simulink model "Arm_cobot"  (Simulink 8.3)
settings: Solver=ode1  StartTime=0.0  StopTime=inf  FixedStep=TA  RelTol=1e-3
PreLoadFcn:
  | startup
  | gui_starter
  | init_starter
PostLoadFcn:
  | init_check
InitFcn:
  | init_starter
undefined symbols (not defined in the file): alphaM, alphaT, Arm7ConLib, Arms2, baseOffset_x, baseOffset_y, baseOffset_z, betaM, betaT, cobotNa, cobotNb, D1, D2, D3, D4, D5, D6, D7, d_FTS_EE_L, d_FTS_EE_R, DD1, DD2, DD3, DD4, DD5, DD6, DD7, Do, Dp, EEL, EER, Fcal_L, Fcal_R, I1, I2, I3, I4, I5, I6, I7, IFL, IFR, impuls2rad_L, impuls2rad_R, Inert_L, Inert_R, KdC, KiC, Ko, Kp, KpC, LTool_L, LTool_R, mEE_L, mEE_R, Mo, Mp, P1, P2, P3 ... (+28)
libraries: sensoray x16, rtai_utilities x11, simulink x2, jr3lib x2, Interface x1
(part 2 of 3)

== system Arm_cobot/Left Arm/PD Joint Control  LEFT/PID Digital Derivative1 ==
  In1 : Inport
  Demux : Demux  Outputs=7
  Mux : Mux  Inputs=7
  PID + digital Derivative1 : Subsystem  AncestorBlock=|  mask(PID(2) Controller){P=P(1), I=I(1), D=D(1), N=N(1)}
      | Arm7lib/PID
      | Digital Derivative/PID +
      | digital Derivative2
      mask prompts: P "Proportional:"; I "Integral:"; D "Derivative:"; N "Derivative divisor(N):"
      mask help:
      | Enter Proportional(P), Integral(I), and Derivative(D) and divisor (N) terms.
      | P+I/s+Ds/(1/Ns+1)
      mask Help: This block implements a PID controller where parameters are entered for the Proportional, Integral and Derivative and divisor terms. Unmask this block to see how it works. The derivative term is implemented using an s/(s/N +1)  transfer function block. Making N large can create a "stiff" system.
      mask Display: disp('PID')
  PID + digital Derivative2 : Subsystem  AncestorBlock=|  mask(PID(2) Controller){P=P(3), I=I(3), D=D(3), N=N(3)}
      | Arm7lib/PID
      | Digital Derivative/PID +
      | digital Derivative2
      mask prompts: P "Proportional:"; I "Integral:"; D "Derivative:"; N "Derivative divisor(N):"
      mask help:
      | Enter Proportional(P), Integral(I), and Derivative(D) and divisor (N) terms.
      | P+I/s+Ds/(1/Ns+1)
      mask Help: This block implements a PID controller where parameters are entered for the Proportional, Integral and Derivative and divisor terms. Unmask this block to see how it works. The derivative term is implemented using an s/(s/N +1)  transfer function block. Making N large can create a "stiff" system.
      mask Display: disp('PID')
  PID + digital Derivative3 : Subsystem  AncestorBlock=|  mask(PID(2) Controller){P=P(2), I=I(2), D=D(2), N=N(2)}
      | Arm7lib/PID
      | Digital Derivative/PID +
      | digital Derivative2
      mask prompts: P "Proportional:"; I "Integral:"; D "Derivative:"; N "Derivative divisor(N):"
      mask help:
      | Enter Proportional(P), Integral(I), and Derivative(D) and divisor (N) terms.
      | P+I/s+Ds/(1/Ns+1)
      mask Help: This block implements a PID controller where parameters are entered for the Proportional, Integral and Derivative and divisor terms. Unmask this block to see how it works. The derivative term is implemented using an s/(s/N +1)  transfer function block. Making N large can create a "stiff" system.
      mask Display: disp('PID')
  PID + digital Derivative4 : Subsystem  AncestorBlock=|  mask(PID(2) Controller){P=P(4), I=I(4), D=D(4), N=N(4)}
      | Arm7lib/PID
      | Digital Derivative/PID +
      | digital Derivative2
      mask prompts: P "Proportional:"; I "Integral:"; D "Derivative:"; N "Derivative divisor(N):"
      mask help:
      | Enter Proportional(P), Integral(I), and Derivative(D) and divisor (N) terms.
      | P+I/s+Ds/(1/Ns+1)
      mask Help: This block implements a PID controller where parameters are entered for the Proportional, Integral and Derivative and divisor terms. Unmask this block to see how it works. The derivative term is implemented using an s/(s/N +1)  transfer function block. Making N large can create a "stiff" system.
      mask Display: disp('PID')
  PID + digital Derivative5 : Subsystem  AncestorBlock=|  mask(PID(2) Controller){P=P(5), I=I(5), D=D(5), N=N(5)}
      | Arm7lib/PID
      | Digital Derivative/PID +
      | digital Derivative2
      mask prompts: P "Proportional:"; I "Integral:"; D "Derivative:"; N "Derivative divisor(N):"
      mask help:
      | Enter Proportional(P), Integral(I), and Derivative(D) and divisor (N) terms.
      | P+I/s+Ds/(1/Ns+1)
      mask Help: This block implements a PID controller where parameters are entered for the Proportional, Integral and Derivative and divisor terms. Unmask this block to see how it works. The derivative term is implemented using an s/(s/N +1)  transfer function block. Making N large can create a "stiff" system.
      mask Display: disp('PID')
  PID + digital Derivative6 : Subsystem  AncestorBlock=|  mask(PID(2) Controller){P=P(6), I=I(6), D=D(6), N=N(6)}
      | Arm7lib/PID
      | Digital Derivative/PID +
      | digital Derivative2
      mask prompts: P "Proportional:"; I "Integral:"; D "Derivative:"; N "Derivative divisor(N):"
      mask help:
      | Enter Proportional(P), Integral(I), and Derivative(D) and divisor (N) terms.
      | P+I/s+Ds/(1/Ns+1)
      mask Help: This block implements a PID controller where parameters are entered for the Proportional, Integral and Derivative and divisor terms. Unmask this block to see how it works. The derivative term is implemented using an s/(s/N +1)  transfer function block. Making N large can create a "stiff" system.
      mask Display: disp('PID')
  PID + digital Derivative7 : Subsystem  AncestorBlock=|  mask(PID(2) Controller){P=P(7), I=I(7), D=D(7), N=N(7)}
      | Arm7lib/PID
      | Digital Derivative/PID +
      | digital Derivative2
      mask prompts: P "Proportional:"; I "Integral:"; D "Derivative:"; N "Derivative divisor(N):"
      mask help:
      | Enter Proportional(P), Integral(I), and Derivative(D) and divisor (N) terms.
      | P+I/s+Ds/(1/Ns+1)
      mask Help: This block implements a PID controller where parameters are entered for the Proportional, Integral and Derivative and divisor terms. Unmask this block to see how it works. The derivative term is implemented using an s/(s/N +1)  transfer function block. Making N large can create a "stiff" system.
      mask Display: disp('PID')
  Out1 : Outport
  wires:
  PID + digital Derivative7/1(Out_1) -> Mux/7
  PID + digital Derivative6/1(Out_1) -> Mux/6
  PID + digital Derivative5/1(Out_1) -> Mux/5
  PID + digital Derivative4/1(Out_1) -> Mux/4
  PID + digital Derivative2/1(Out_1) -> Mux/3
  PID + digital Derivative3/1(Out_1) -> Mux/2
  Demux/7 -> PID + digital Derivative7/1(In_1)
  Demux/6 -> PID + digital Derivative6/1(In_1)
  Demux/5 -> PID + digital Derivative5/1(In_1)
  Demux/4 -> PID + digital Derivative4/1(In_1)
  Demux/3 -> PID + digital Derivative2/1(In_1)
  Demux/2 -> PID + digital Derivative3/1(In_1)
  Mux/1 -> Out1/1
  PID + digital Derivative1/1(Out_1) -> Mux/1
  Demux/1 -> PID + digital Derivative1/1(In_1)
  In1/1 -> Demux/1

== system Arm_cobot/Left Arm/Switch between position control for Init position and regular controller/BackToInit1 ==
  JointAngles [rad] : Inport
  Clock : Clock
  "InitialJointAngles " : Constant  Value=qIL
  InitialPosition : S-Function  FunctionName=BackToInitJointSpace  EnableBusSupport=off
  Integrator : Integrator  InitialConditionSource=external
  Mux : Mux  Inputs=3
  Zeros : Constant  Value=zeros(1,7)
  q [rad] : Outport
  wires:
  Clock/1 -> Mux/3
  Mux/1 -> InitialPosition/1
  JointAngles [rad]/1 -> Integrator/2
  Zeros/1 -> Integrator/1
  Integrator/1 -> Mux/1
  InitialPosition/1 -> q [rad]/1
  "InitialJointAngles "/1 -> Mux/2

== system Arm_cobot/Right Arm/Feedforward/second  derivative ==
  q : Inport
  2ndDerivative3Points : MATLAB Function  TreatAsAtomicUnit=on
  Constant : Constant  Value=10*ones(1,7)
  Constant1 : Constant  Value=-10*ones(1,7)
  Memory : Memory
  Memory1 : Memory
  Rate Limiter Dynamic : simulink/Discontinuities/Rate Limiter Dynamic
  qDotDot : Outport
  wires:
  q/1 -> Memory/1, 2ndDerivative3Points/1(u0)
  Memory/1 -> Memory1/1, 2ndDerivative3Points/2(u1)
  Memory1/1 -> 2ndDerivative3Points/3(u2)
  Constant/1 -> Rate Limiter Dynamic/1
  Constant1/1 -> Rate Limiter Dynamic/3
  Rate Limiter Dynamic/1 -> qDotDot/1
  2ndDerivative3Points/1(y) -> Rate Limiter Dynamic/2

== system Arm_cobot/Right Arm/ForceControl/Subsystem ==
  In1 : Inport
  reset : Inport  Port=2
  Demux : Demux  Outputs=6
  Mux : Mux  Inputs=6
  PII : Subsystem  AncestorBlock=|  mask(PID(2) Controller){P=PF(1), I=IF(1), S=SF(1)}
      | Arm7lib/PID
      | Digital Derivative/PID +
      | digital Derivative2
      mask prompts: P "Proportional:"; I "Integral:"; S "Saturation:"
      mask help:
      | Enter Proportional(P), Integral(I), and Derivative(D) and divisor (N) terms.
      | P+I/s+Ds/(1/Ns+1)
      mask Help: This block implements a PID controller where parameters are entered for the Proportional, Integral and Derivative and divisor terms. Unmask this block to see how it works. The derivative term is implemented using an s/(s/N +1)  transfer function block. Making N large can create a "stiff" system.
      mask Display: disp('PI')
  PII1 : Subsystem  AncestorBlock=|  mask(PID(2) Controller){P=PF(2), I=IF(2), S=SF(2)}
      | Arm7lib/PID
      | Digital Derivative/PID +
      | digital Derivative2
      mask prompts: P "Proportional:"; I "Integral:"; S "Saturation:"
      mask help:
      | Enter Proportional(P), Integral(I), and Derivative(D) and divisor (N) terms.
      | P+I/s+Ds/(1/Ns+1)
      mask Help: This block implements a PID controller where parameters are entered for the Proportional, Integral and Derivative and divisor terms. Unmask this block to see how it works. The derivative term is implemented using an s/(s/N +1)  transfer function block. Making N large can create a "stiff" system.
      mask Display: disp('PI')
  PII2 : Subsystem  AncestorBlock=|  mask(PID(2) Controller){P=PF(3), I=IF(3), S=SF(3)}
      | Arm7lib/PID
      | Digital Derivative/PID +
      | digital Derivative2
      mask prompts: P "Proportional:"; I "Integral:"; S "Saturation:"
      mask help:
      | Enter Proportional(P), Integral(I), and Derivative(D) and divisor (N) terms.
      | P+I/s+Ds/(1/Ns+1)
      mask Help: This block implements a PID controller where parameters are entered for the Proportional, Integral and Derivative and divisor terms. Unmask this block to see how it works. The derivative term is implemented using an s/(s/N +1)  transfer function block. Making N large can create a "stiff" system.
      mask Display: disp('PI')
  PII3 : Subsystem  AncestorBlock=|  mask(PID(2) Controller){P=PF(4), I=IF(4), S=SF(4)}
      | Arm7lib/PID
      | Digital Derivative/PID +
      | digital Derivative2
      mask prompts: P "Proportional:"; I "Integral:"; S "Saturation:"
      mask help:
      | Enter Proportional(P), Integral(I), and Derivative(D) and divisor (N) terms.
      | P+I/s+Ds/(1/Ns+1)
      mask Help: This block implements a PID controller where parameters are entered for the Proportional, Integral and Derivative and divisor terms. Unmask this block to see how it works. The derivative term is implemented using an s/(s/N +1)  transfer function block. Making N large can create a "stiff" system.
      mask Display: disp('PI')
  PII4 : Subsystem  AncestorBlock=|  mask(PID(2) Controller){P=PF(5), I=IF(5), S=SF(5)}
      | Arm7lib/PID
      | Digital Derivative/PID +
      | digital Derivative2
      mask prompts: P "Proportional:"; I "Integral:"; S "Saturation:"
      mask help:
      | Enter Proportional(P), Integral(I), and Derivative(D) and divisor (N) terms.
      | P+I/s+Ds/(1/Ns+1)
      mask Help: This block implements a PID controller where parameters are entered for the Proportional, Integral and Derivative and divisor terms. Unmask this block to see how it works. The derivative term is implemented using an s/(s/N +1)  transfer function block. Making N large can create a "stiff" system.
      mask Display: disp('PI')
  PII5 : Subsystem  AncestorBlock=|  mask(PID(2) Controller){P=PF(6), I=IF(6), S=SF(6)}
      | Arm7lib/PID
      | Digital Derivative/PID +
      | digital Derivative2
      mask prompts: P "Proportional:"; I "Integral:"; S "Saturation:"
      mask help:
      | Enter Proportional(P), Integral(I), and Derivative(D) and divisor (N) terms.
      | P+I/s+Ds/(1/Ns+1)
      mask Help: This block implements a PID controller where parameters are entered for the Proportional, Integral and Derivative and divisor terms. Unmask this block to see how it works. The derivative term is implemented using an s/(s/N +1)  transfer function block. Making N large can create a "stiff" system.
      mask Display: disp('PI')
  Out1 : Outport
  wires:
  In1/1 -> Demux/1
  Demux/1 -> PII/1(In_1)
  Demux/2 -> PII1/1(In_1)
  Demux/3 -> PII2/1(In_1)
  Demux/5 -> PII4/1(In_1)
  PII/1(Out_1) -> Mux/1
  PII1/1(Out_1) -> Mux/2
  PII2/1(Out_1) -> Mux/3
  PII3/1(Out_1) -> Mux/4
  PII4/1(Out_1) -> Mux/5
  PII5/1(Out_1) -> Mux/6
  Mux/1 -> Out1/1
  Demux/6 -> PII5/1(In_1)
  reset/1 -> PII/2(reset), PII1/2(reset), PII2/2(reset), PII3/2(reset), PII5/2(reset), PII4/2(reset)
  Demux/4 -> PII3/1(In_1)

== system Arm_cobot/Right Arm/ForceControl/lowpass ==
  fLc : Inport
  Demux : Demux  Outputs=6
  Discrete Filter{,1..5} (6 alike) : DiscreteFilter  Numerator=[0.1 0.1 0.1 0.1 0.1 0.1 0.1 0.1 0.1 0.1]  Denominator=[1]
  Mux2 : Mux  Inputs=6
  Rate Transition3 : RateTransition  X0=-1
  smoothed : Outport
  wires:
  Discrete Filter/1 -> Mux2/1
  Demux/1 -> Discrete Filter/1
  Demux/2 -> Discrete Filter1/1
  Demux/3 -> Discrete Filter2/1
  Demux/4 -> Discrete Filter3/1
  Demux/5 -> Discrete Filter4/1
  Demux/6 -> Discrete Filter5/1
  Discrete Filter1/1 -> Mux2/2
  Discrete Filter3/1 -> Mux2/4
  Discrete Filter4/1 -> Mux2/5
  Discrete Filter5/1 -> Mux2/6
  Mux2/1 -> smoothed/1
  fLc/1 -> Rate Transition3/1
  Rate Transition3/1 -> Demux/1
  Discrete Filter2/1 -> Mux2/3

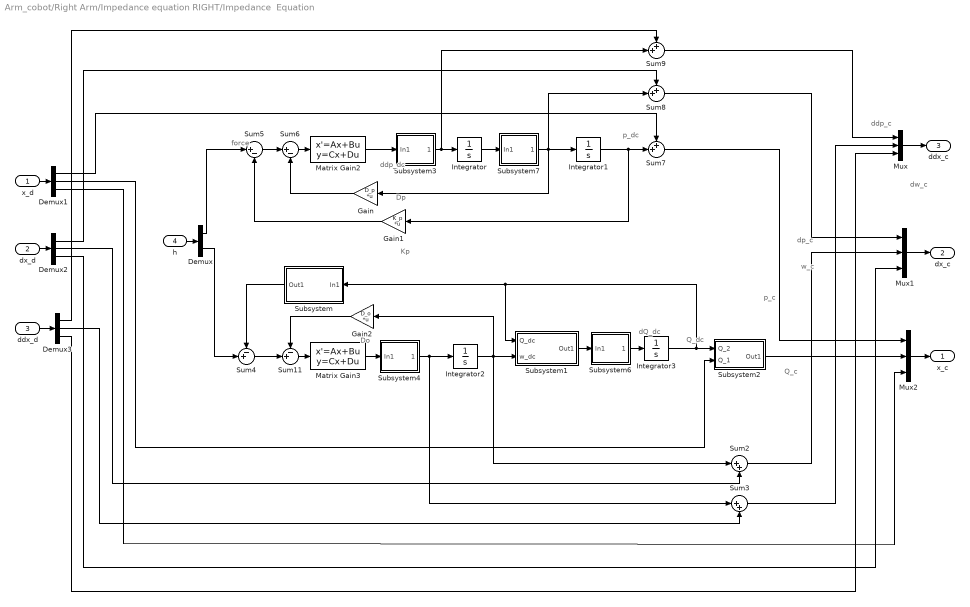
== system Arm_cobot/Right Arm/Impedance equation RIGHT/Impedance  Equation ==
  note: Do
  note: Dp
  note: Kp
  note: p_dc
  note: ddp_dc
  note: force
  note: p_c
  note: dp_c
  note: ddp_c
  note: dQ_dc
  note: Q_dc
  note: dw_c
  note: w_c
  note: Q_c
  x_d : Inport
  dx_d : Inport  Port=2
  ddx_d : Inport  Port=3
  h : Inport  Port=4
  Demux : Demux  Outputs=[3,3]
  Demux1 : Demux  Outputs=[3, 4, 1]
  Demux2 : Demux  Outputs=[3,3,1]
  Demux3 : Demux  Outputs=[3,3,1]
  Gain : Gain  Gain=D_p  Multiplication=Matrix(K*u)  OutDataTypeStr=Inherit: Same as input  ParamDataTypeStr=Inherit: Same as input
  Gain1 : Gain  Gain=K_p  Multiplication=Matrix(K*u)  OutDataTypeStr=Inherit: Same as input  ParamDataTypeStr=Inherit: Same as input
  Gain2 : Gain  Gain=D_o  Multiplication=Matrix(K*u)  OutDataTypeStr=Inherit: Same as input  ParamDataTypeStr=Inherit: Same as input
  Integrator : Integrator  InitialCondition=[0 0 0]
  Integrator1 : Integrator  InitialCondition=[0 0 0]
  Integrator2 : Integrator  InitialCondition=[0 0 0]
  Integrator3 : Integrator  InitialCondition=[1 0 0 0]
  Matrix Gain2 : StateSpace  A=[]  B=[]  C=[]  D=K  X0=0  mask(Matrix Gain){K=inv(M_p)}
      mask prompts: K "Gain matrix:"
      mask help: Matrix Gain.
      mask Help: Multiplies input vector by entered matrix to produce output vector (y=Au).
      mask Display: disp('inv(Mp)')
  Matrix Gain3 : StateSpace  A=[]  B=[]  C=[]  D=K  X0=0  mask(Matrix Gain){K=inv(M_o)}
      mask prompts: K "Gain matrix:"
      mask help: Matrix Gain.
      mask Help: Multiplies input vector by entered matrix to produce output vector (y=Au).
      mask Display: disp('inv(Mo)')
  Mux : Mux  Inputs=3
  Mux1 : Mux  Inputs=3
  Mux2 : Mux  Inputs=[3,4,1]
  Subsystem : Subsystem
      mask Display: disp('2*tr(E)*Ko')
  Subsystem1 : Subsystem
      mask Display: disp('Quaternion\n Propagation')
  Subsystem2 : Subsystem
      mask Display: disp('Qproduct')
  Subsystem3 : Subsystem
  Subsystem4 : Subsystem
  Subsystem6 : Subsystem
  Subsystem7 : Subsystem
  Sum11 : Sum  Inputs=-+|  SaturateOnIntegerOverflow=on  InputSameDT=on  OutDataTypeStr=Inherit: Same as first input
  Sum2 : Sum  Inputs=|++  SaturateOnIntegerOverflow=on  InputSameDT=on  OutDataTypeStr=Inherit: Same as first input
  Sum3 : Sum  Inputs=|++  SaturateOnIntegerOverflow=on  InputSameDT=on  OutDataTypeStr=Inherit: Same as first input
  Sum4 : Sum  Inputs=-+|  SaturateOnIntegerOverflow=on  InputSameDT=on  OutDataTypeStr=Inherit: Same as first input
  Sum5 : Sum  Inputs=|+-  SaturateOnIntegerOverflow=on  InputSameDT=on  OutDataTypeStr=Inherit: Same as first input
  Sum6 : Sum  Inputs=|+-  SaturateOnIntegerOverflow=on  InputSameDT=on  OutDataTypeStr=Inherit: Same as first input
  Sum7 : Sum  Inputs=++|  SaturateOnIntegerOverflow=on  InputSameDT=on  OutDataTypeStr=Inherit: Same as first input
  Sum8 : Sum  Inputs=++|  SaturateOnIntegerOverflow=on  InputSameDT=on  OutDataTypeStr=Inherit: Same as first input
  Sum9 : Sum  Inputs=++|  SaturateOnIntegerOverflow=on  InputSameDT=on  OutDataTypeStr=Inherit: Same as first input
  x_c : Outport
  dx_c : Outport  Port=2
  ddx_c : Outport  Port=3
  wires:
  Demux1/2 -> Subsystem2/2(Q_1)
  Subsystem2/1(Out1) -> Mux2/2
  Mux2/1 -> x_c/1
  Demux3/2 -> Sum3/2
  Demux3/3 -> Mux/3
  Mux1/1 -> dx_c/1
  Demux1/3 -> Mux2/3
  Demux2/3 -> Mux1/3
  Gain1/1 -> Sum5/2
  Gain/1 -> Sum6/2
  Subsystem1/1(Out1) -> Subsystem6/1(In1)
  Subsystem/1(Out1) -> Sum4/1
  Sum8/1 -> Mux1/1
  Sum6/1 -> Matrix Gain2/1
  Integrator1/1 -> Sum7/2, Gain1/1
  Sum5/1 -> Sum6/1
  Integrator/1 -> Subsystem7/1(In1)
  Integrator2/1 -> Subsystem1/2(w_dc), Gain2/1, Sum2/1
  Matrix Gain3/1 -> Subsystem4/1(In1)
  Sum2/1 -> Mux1/2
  h/1 -> Demux/1
  Sum9/1 -> Mux/1
  Mux/1 -> ddx_c/1
  Gain2/1 -> Sum11/1
  Sum11/1 -> Matrix Gain3/1
  Sum4/1 -> Sum11/2
  x_d/1 -> Demux1/1
  dx_d/1 -> Demux2/1
  ddx_d/1 -> Demux3/1
  Demux1/1 -> Sum7/1
  Demux2/2 -> Sum2/2
  Demux2/1 -> Sum8/1
  Demux3/1 -> Sum9/1
  Sum3/1 -> Mux/2
  Integrator3/1 -> Subsystem2/1(Q_2), Subsystem/1(In1), Subsystem1/1(Q_dc)
  Sum7/1 -> Mux2/1
  Demux/1 -> Sum5/1
  Demux/2 -> Sum4/2
  Subsystem3/1(Out1) -> Integrator/1, Sum9/2
  Matrix Gain2/1 -> Subsystem3/1(In1)
  Subsystem6/1(Out1) -> Integrator3/1
  Subsystem7/1(Out1) -> Sum8/2, Gain/1, Integrator1/1
  Subsystem4/1(Out1) -> Sum3/1, Integrator2/1

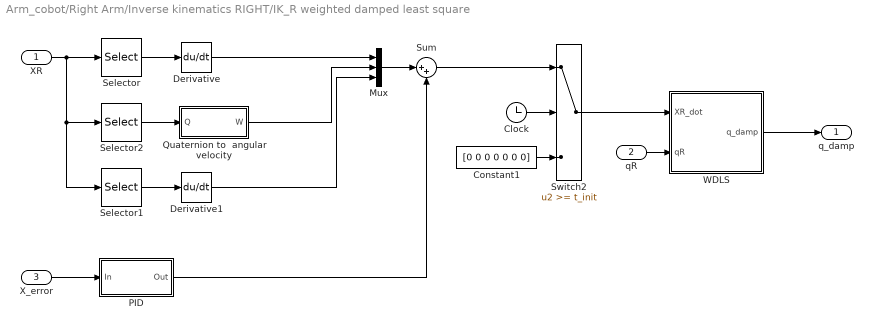
== system Arm_cobot/Right Arm/Inverse kinematics RIGHT/IK_R weighted damped least square ==
  XR : Inport
  qR : Inport  Port=2
  X_error : Inport  Port=3
  Clock : Clock
  Constant1 : Constant  Value=[0 0 0 0 0 0 0]
  Derivative : Derivative
  Derivative1 : Derivative
  Mux : Mux  Inputs=3
  PID : Subsystem
  Quaternion to  angular velocity : Subsystem
  Selector : Selector  InputPortWidth=8  Indices=[1:3]
  Selector1 : Selector  InputPortWidth=8  Indices=[8]
  Selector2 : Selector  InputPortWidth=8  Indices=[4:7]
  Sum : Sum  Inputs=|++
  Switch2 : Switch  Threshold=t_init  SaturateOnIntegerOverflow=on  InputSameDT=on
  WDLS : Subsystem
  q_damp : Outport
  wires:
  XR/1 -> Selector/1, Selector2/1, Selector1/1
  qR/1 -> WDLS/2(qR)
  X_error/1 -> PID/1(In)
  WDLS/1(q_damp) -> q_damp/1
  Derivative1/1 -> Mux/3
  Derivative/1 -> Mux/1
  Selector2/1 -> Quaternion to  angular velocity/1(Q)
  Selector/1 -> Derivative/1
  Switch2/1 -> WDLS/1(XR_dot)
  Quaternion to  angular velocity/1(W) -> Mux/2
  Constant1/1 -> Switch2/3
  Clock/1 -> Switch2/2
  Selector1/1 -> Derivative1/1
  Mux/1 -> Sum/1
  Sum/1 -> Switch2/1
  PID/1(Out) -> Sum/2

== system Arm_cobot/Right Arm/Inverse kinematics RIGHT/pose error in task space ==
  x_d : Inport
  x_m : Inport  Port=2
  qR : Inport  Port=3
  Embedded MATLAB Function : MATLAB Function  TreatAsAtomicUnit=on
  Mux1 : Mux  Inputs=2
  S-Function : S-Function  FunctionName=PoseError_S  EnableBusSupport=off
  X_error : Outport
  wires:
  Mux1/1 -> S-Function/1
  x_m/1 -> Mux1/2
  x_d/1 -> Mux1/1
  S-Function/1 -> Embedded MATLAB Function/1(errIn)
  Embedded MATLAB Function/1(errOut) -> X_error/1
  qR/1 -> Embedded MATLAB Function/2(qIn)

== system Arm_cobot/Right Arm/PD Joint Control  RIGHT/PID Digital Derivative1 ==
  In1 : Inport
  Demux : Demux  Outputs=7
  Mux : Mux  Inputs=7
  PID + digital Derivative1 : Subsystem  AncestorBlock=|  mask(PID(2) Controller){P=P(1), I=I(1), D=D(1), N=N(1)}
      | Arm7lib/PID
      | Digital Derivative/PID +
      | digital Derivative2
      mask prompts: P "Proportional:"; I "Integral:"; D "Derivative:"; N "Derivative divisor(N):"
      mask help:
      | Enter Proportional(P), Integral(I), and Derivative(D) and divisor (N) terms.
      | P+I/s+Ds/(1/Ns+1)
      mask Help: This block implements a PID controller where parameters are entered for the Proportional, Integral and Derivative and divisor terms. Unmask this block to see how it works. The derivative term is implemented using an s/(s/N +1)  transfer function block. Making N large can create a "stiff" system.
      mask Display: disp('PID')
  PID + digital Derivative2 : Subsystem  AncestorBlock=|  mask(PID(2) Controller){P=P(3), I=I(3), D=D(3), N=N(3)}
      | Arm7lib/PID
      | Digital Derivative/PID +
      | digital Derivative2
      mask prompts: P "Proportional:"; I "Integral:"; D "Derivative:"; N "Derivative divisor(N):"
      mask help:
      | Enter Proportional(P), Integral(I), and Derivative(D) and divisor (N) terms.
      | P+I/s+Ds/(1/Ns+1)
      mask Help: This block implements a PID controller where parameters are entered for the Proportional, Integral and Derivative and divisor terms. Unmask this block to see how it works. The derivative term is implemented using an s/(s/N +1)  transfer function block. Making N large can create a "stiff" system.
      mask Display: disp('PID')
  PID + digital Derivative3 : Subsystem  AncestorBlock=|  mask(PID(2) Controller){P=P(2), I=I(2), D=D(2), N=N(2)}
      | Arm7lib/PID
      | Digital Derivative/PID +
      | digital Derivative2
      mask prompts: P "Proportional:"; I "Integral:"; D "Derivative:"; N "Derivative divisor(N):"
      mask help:
      | Enter Proportional(P), Integral(I), and Derivative(D) and divisor (N) terms.
      | P+I/s+Ds/(1/Ns+1)
      mask Help: This block implements a PID controller where parameters are entered for the Proportional, Integral and Derivative and divisor terms. Unmask this block to see how it works. The derivative term is implemented using an s/(s/N +1)  transfer function block. Making N large can create a "stiff" system.
      mask Display: disp('PID')
  PID + digital Derivative4 : Subsystem  AncestorBlock=|  mask(PID(2) Controller){P=P(4), I=I(4), D=D(4), N=N(4)}
      | Arm7lib/PID
      | Digital Derivative/PID +
      | digital Derivative2
      mask prompts: P "Proportional:"; I "Integral:"; D "Derivative:"; N "Derivative divisor(N):"
      mask help:
      | Enter Proportional(P), Integral(I), and Derivative(D) and divisor (N) terms.
      | P+I/s+Ds/(1/Ns+1)
      mask Help: This block implements a PID controller where parameters are entered for the Proportional, Integral and Derivative and divisor terms. Unmask this block to see how it works. The derivative term is implemented using an s/(s/N +1)  transfer function block. Making N large can create a "stiff" system.
      mask Display: disp('PID')
  PID + digital Derivative5 : Subsystem  AncestorBlock=|  mask(PID(2) Controller){P=P(5), I=I(5), D=D(5), N=N(5)}
      | Arm7lib/PID
      | Digital Derivative/PID +
      | digital Derivative2
      mask prompts: P "Proportional:"; I "Integral:"; D "Derivative:"; N "Derivative divisor(N):"
      mask help:
      | Enter Proportional(P), Integral(I), and Derivative(D) and divisor (N) terms.
      | P+I/s+Ds/(1/Ns+1)
      mask Help: This block implements a PID controller where parameters are entered for the Proportional, Integral and Derivative and divisor terms. Unmask this block to see how it works. The derivative term is implemented using an s/(s/N +1)  transfer function block. Making N large can create a "stiff" system.
      mask Display: disp('PID')
  PID + digital Derivative6 : Subsystem  AncestorBlock=|  mask(PID(2) Controller){P=P(6), I=I(6), D=D(6), N=N(6)}
      | Arm7lib/PID
      | Digital Derivative/PID +
      | digital Derivative2
      mask prompts: P "Proportional:"; I "Integral:"; D "Derivative:"; N "Derivative divisor(N):"
      mask help:
      | Enter Proportional(P), Integral(I), and Derivative(D) and divisor (N) terms.
      | P+I/s+Ds/(1/Ns+1)
      mask Help: This block implements a PID controller where parameters are entered for the Proportional, Integral and Derivative and divisor terms. Unmask this block to see how it works. The derivative term is implemented using an s/(s/N +1)  transfer function block. Making N large can create a "stiff" system.
      mask Display: disp('PID')
  PID + digital Derivative7 : Subsystem  AncestorBlock=|  mask(PID(2) Controller){P=P(7), I=I(7), D=D(7), N=N(7)}
      | Arm7lib/PID
      | Digital Derivative/PID +
      | digital Derivative2
      mask prompts: P "Proportional:"; I "Integral:"; D "Derivative:"; N "Derivative divisor(N):"
      mask help:
      | Enter Proportional(P), Integral(I), and Derivative(D) and divisor (N) terms.
      | P+I/s+Ds/(1/Ns+1)
      mask Help: This block implements a PID controller where parameters are entered for the Proportional, Integral and Derivative and divisor terms. Unmask this block to see how it works. The derivative term is implemented using an s/(s/N +1)  transfer function block. Making N large can create a "stiff" system.
      mask Display: disp('PID')
  Out1 : Outport
  wires:
  PID + digital Derivative7/1(Out_1) -> Mux/7
  PID + digital Derivative6/1(Out_1) -> Mux/6
  PID + digital Derivative5/1(Out_1) -> Mux/5
  PID + digital Derivative4/1(Out_1) -> Mux/4
  PID + digital Derivative2/1(Out_1) -> Mux/3
  PID + digital Derivative3/1(Out_1) -> Mux/2
  Demux/7 -> PID + digital Derivative7/1(In_1)
  Demux/6 -> PID + digital Derivative6/1(In_1)
  Demux/5 -> PID + digital Derivative5/1(In_1)
  Demux/4 -> PID + digital Derivative4/1(In_1)
  Demux/3 -> PID + digital Derivative2/1(In_1)
  Demux/2 -> PID + digital Derivative3/1(In_1)
  Mux/1 -> Out1/1
  PID + digital Derivative1/1(Out_1) -> Mux/1
  Demux/1 -> PID + digital Derivative1/1(In_1)
  In1/1 -> Demux/1

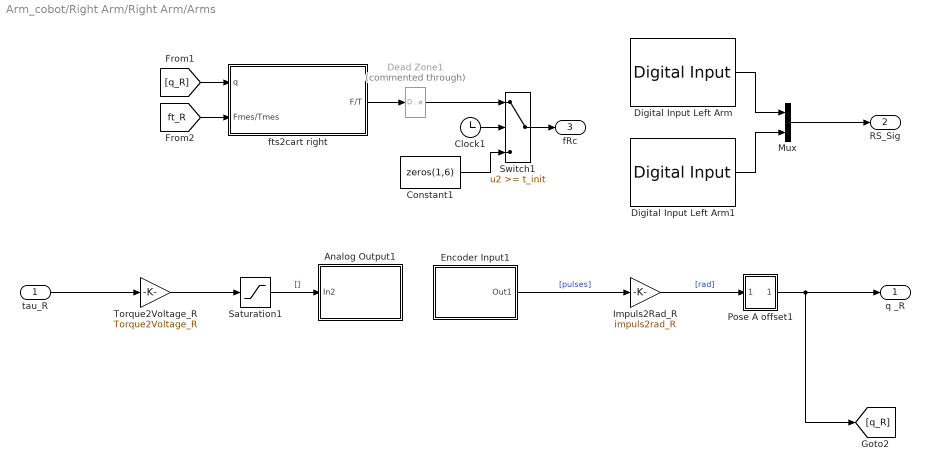
== system Arm_cobot/Right Arm/Right Arm/Arms ==
  tau_R : Inport
  Analog Output1 : Subsystem
      mask Display: disp('DAC')
  Clock1 : Clock
  Constant1 : Constant  Value=zeros(1,6)
  Dead Zone1 : DeadZone  Commented=through  LowerValue=[-2.5 -2.5 -2.5 -0.25 -0.25 -0.25]  UpperValue=[2.5 2.5 2.5 0.25 0.25 0.25]  SaturateOnIntegerOverflow=on
  Digital Input Left Arm : sensoray/Digital Input  BoardNumber=0  Channels=[35 34 33 32]  SampleTime=simget(bdroot,'FixedStep')
  Digital Input Left Arm1 : sensoray/Digital Input  BoardNumber=1  Channels=[35 34 33]  SampleTime=simget(bdroot,'FixedStep')
  Encoder Input1 : Subsystem
      mask Display: disp('ENC')
  Impuls2Rad_R : Gain  Gain=impuls2rad_R  SaturateOnIntegerOverflow=on  OutDataTypeStr=Inherit: Same as input  ParamDataTypeStr=Inherit: Same as input
  Mux : Mux  Inputs=2
  Pose A offset1 : Subsystem
      mask Display: disp('Pose\nOffset')
  Saturation1 : Saturate  UpperLimit=umaxR  LowerLimit=uminR
  Switch1 : Switch  Threshold=t_init  SaturateOnIntegerOverflow=on  InputSameDT=on
  Torque2Voltage_R : Gain  Gain=Torque2Voltage_R  SaturateOnIntegerOverflow=on  OutDataTypeStr=Inherit: Same as input  ParamDataTypeStr=Inherit: Same as input
  fts2cart right : Subsystem  mask(Transformation of measured force/torque of FT-sensor into the Newtonian frame){MEE=mEE_R, LEE=d_FTS_EE_R, OFFbee=p_EE_o_R, Fcal=Fcal_R, Tcal=Tcal_R, LTCP=LTool_R}
      mask prompts: MEE "Endeffector mass"; LEE "Distance of endeffector to FT-sensor coordinate system"; OFFbee "Location of center of gravity of the endeffector in endeffector coordinate system"; Fcal "Force acting at the FT-sensor  in the moment of calibration, given in FTS coordinate system"; Tcal "Torque acting at the FT-sensor in the moment of calibration given in the FTS coordinate system"; LTCP "Location of tool center point (point at which the master motion will be mapped) given in the FT-sensor coordinate system"
      mask help: Transforms the measured force/torque given in the FT-sensor coordinate system into the Newtonian frame. Additionally the endeffector mass and inertia are compensated.
  q _R : Outport
  RS_Sig : Outport  Port=2
  fRc : Outport  Port=3
  wires:
  Pose A offset1/1(out) -> q _R/1, [q_R]
  Encoder Input1/1(Out1) -> Impuls2Rad_R/1  "[pulses]"
  Impuls2Rad_R/1 -> Pose A offset1/1(in)  "[rad]"
  Saturation1/1 -> Analog Output1/1(In2)  "[]"
  Torque2Voltage_R/1 -> Saturation1/1
  fts2cart right/1(F/T) -> Dead Zone1/1
  [q_R] -> fts2cart right/1(q)
  Dead Zone1/1 -> Switch1/1
  Switch1/1 -> fRc/1
  Clock1/1 -> Switch1/2
  Constant1/1 -> Switch1/3
  Mux/1 -> RS_Sig/1
  Digital Input Left Arm/1 -> Mux/1
  Digital Input Left Arm1/1 -> Mux/2
  tau_R/1 -> Torque2Voltage_R/1
  [ft_R] -> fts2cart right/2(Fmes/Tmes)

== system Arm_cobot/Right Arm/Switch between position control for Init position and regular controller/BackToInit1 ==
  JointAngles [rad] : Inport
  Clock : Clock
  "InitialJointAngles " : Constant  Value=qIR
  InitialPosition : S-Function  FunctionName=BackToInitJointSpace  EnableBusSupport=off
  Integrator : Integrator  InitialConditionSource=external
  Mux : Mux  Inputs=3
  Zeros : Constant  Value=zeros(1,7)
  q [rad] : Outport
  wires:
  Clock/1 -> Mux/3
  Mux/1 -> InitialPosition/1
  JointAngles [rad]/1 -> Integrator/2
  Zeros/1 -> Integrator/1
  Integrator/1 -> Mux/1
  InitialPosition/1 -> q [rad]/1
  "InitialJointAngles "/1 -> Mux/2

== system Arm_cobot/Left Arm/ForceControl/Subsystem/PII ==
  In_1 : Inport
  reset : Inport  Port=2
  Integrator : Integrator  ExternalReset=falling  UpperSaturationLimit=S  LowerSaturationLimit=-S
  Proportional : Gain  Gain=P  SaturateOnIntegerOverflow=on  OutDataTypeStr=Inherit: Same as input  ParamDataTypeStr=Inherit: Same as input
  Saturation : Saturate  UpperLimit=S  LowerLimit=-S
  Sum : Sum  SaturateOnIntegerOverflow=on  InputSameDT=on  OutDataTypeStr=Inherit: Same as first input
  Sum1 : Sum  Inputs=-+|
  Sum2 : Sum  Inputs=|++
  Out_1 : Outport  InitialOutput=0
  wires:
  Proportional/1 -> Sum/1
  Integrator/1 -> Sum/2
  Sum/1 -> Sum1/1, Saturation/1
  Sum2/1 -> Integrator/1
  In_1/1 -> Sum2/1, Proportional/1
  Saturation/1 -> Sum1/2, Out_1/1
  Sum1/1 -> Sum2/2
  reset/1 -> Integrator/2

== system Arm_cobot/Left Arm/ForceControl/Subsystem/PII1 ==
  In_1 : Inport
  reset : Inport  Port=2
  Integrator : Integrator  ExternalReset=falling  UpperSaturationLimit=S  LowerSaturationLimit=-S
  Proportional : Gain  Gain=P  SaturateOnIntegerOverflow=on  OutDataTypeStr=Inherit: Same as input  ParamDataTypeStr=Inherit: Same as input
  Saturation : Saturate  UpperLimit=S  LowerLimit=-S
  Sum : Sum  SaturateOnIntegerOverflow=on  InputSameDT=on  OutDataTypeStr=Inherit: Same as first input
  Sum1 : Sum  Inputs=-+|
  Sum2 : Sum  Inputs=|++
  Out_1 : Outport  InitialOutput=0
  wires:
  Proportional/1 -> Sum/1
  Integrator/1 -> Sum/2
  Sum/1 -> Sum1/1, Saturation/1
  Sum2/1 -> Integrator/1
  In_1/1 -> Sum2/1, Proportional/1
  Saturation/1 -> Sum1/2, Out_1/1
  Sum1/1 -> Sum2/2
  reset/1 -> Integrator/2

== system Arm_cobot/Left Arm/ForceControl/Subsystem/PII2 ==
  In_1 : Inport
  reset : Inport  Port=2
  Integrator : Integrator  ExternalReset=falling  UpperSaturationLimit=S  LowerSaturationLimit=-S
  Proportional : Gain  Gain=P  SaturateOnIntegerOverflow=on  OutDataTypeStr=Inherit: Same as input  ParamDataTypeStr=Inherit: Same as input
  Saturation : Saturate  UpperLimit=S  LowerLimit=-S
  Sum : Sum  SaturateOnIntegerOverflow=on  InputSameDT=on  OutDataTypeStr=Inherit: Same as first input
  Sum1 : Sum  Inputs=-+|
  Sum2 : Sum  Inputs=|++
  Out_1 : Outport  InitialOutput=0
  wires:
  Proportional/1 -> Sum/1
  Integrator/1 -> Sum/2
  Sum/1 -> Sum1/1, Saturation/1
  Sum2/1 -> Integrator/1
  In_1/1 -> Sum2/1, Proportional/1
  Saturation/1 -> Sum1/2, Out_1/1
  Sum1/1 -> Sum2/2
  reset/1 -> Integrator/2

== system Arm_cobot/Left Arm/ForceControl/Subsystem/PII3 ==
  In_1 : Inport
  reset : Inport  Port=2
  Integrator : Integrator  ExternalReset=falling  UpperSaturationLimit=S  LowerSaturationLimit=-S
  Proportional : Gain  Gain=P  SaturateOnIntegerOverflow=on  OutDataTypeStr=Inherit: Same as input  ParamDataTypeStr=Inherit: Same as input
  Saturation : Saturate  UpperLimit=S  LowerLimit=-S
  Sum : Sum  SaturateOnIntegerOverflow=on  InputSameDT=on  OutDataTypeStr=Inherit: Same as first input
  Sum1 : Sum  Inputs=-+|
  Sum2 : Sum  Inputs=|++
  Out_1 : Outport  InitialOutput=0
  wires:
  Proportional/1 -> Sum/1
  Integrator/1 -> Sum/2
  Sum/1 -> Sum1/1, Saturation/1
  Sum2/1 -> Integrator/1
  In_1/1 -> Sum2/1, Proportional/1
  Saturation/1 -> Sum1/2, Out_1/1
  Sum1/1 -> Sum2/2
  reset/1 -> Integrator/2

== system Arm_cobot/Left Arm/ForceControl/Subsystem/PII4 ==
  In_1 : Inport
  reset : Inport  Port=2
  Integrator : Integrator  ExternalReset=falling  UpperSaturationLimit=S  LowerSaturationLimit=-S
  Proportional : Gain  Gain=P  SaturateOnIntegerOverflow=on  OutDataTypeStr=Inherit: Same as input  ParamDataTypeStr=Inherit: Same as input
  Saturation : Saturate  UpperLimit=S  LowerLimit=-S
  Sum : Sum  SaturateOnIntegerOverflow=on  InputSameDT=on  OutDataTypeStr=Inherit: Same as first input
  Sum1 : Sum  Inputs=-+|
  Sum2 : Sum  Inputs=|++
  Out_1 : Outport  InitialOutput=0
  wires:
  Proportional/1 -> Sum/1
  Integrator/1 -> Sum/2
  Sum/1 -> Sum1/1, Saturation/1
  Sum2/1 -> Integrator/1
  In_1/1 -> Sum2/1, Proportional/1
  Saturation/1 -> Sum1/2, Out_1/1
  Sum1/1 -> Sum2/2
  reset/1 -> Integrator/2

== system Arm_cobot/Left Arm/ForceControl/Subsystem/PII5 ==
  In_1 : Inport
  reset : Inport  Port=2
  Integrator : Integrator  ExternalReset=falling  UpperSaturationLimit=S  LowerSaturationLimit=-S
  Proportional : Gain  Gain=P  SaturateOnIntegerOverflow=on  OutDataTypeStr=Inherit: Same as input  ParamDataTypeStr=Inherit: Same as input
  Saturation : Saturate  UpperLimit=S  LowerLimit=-S
  Sum : Sum  SaturateOnIntegerOverflow=on  InputSameDT=on  OutDataTypeStr=Inherit: Same as first input
  Sum1 : Sum  Inputs=-+|
  Sum2 : Sum  Inputs=|++
  Out_1 : Outport  InitialOutput=0
  wires:
  Proportional/1 -> Sum/1
  Integrator/1 -> Sum/2
  Sum/1 -> Sum1/1, Saturation/1
  Sum2/1 -> Integrator/1
  In_1/1 -> Sum2/1, Proportional/1
  Saturation/1 -> Sum1/2, Out_1/1
  Sum1/1 -> Sum2/2
  reset/1 -> Integrator/2

== system Arm_cobot/Left Arm/Impedance equation LEFT/Impedance  Equation/Subsystem ==
  In1 : Inport
  Demux : Demux  Outputs=[1,3]
  Demux1 : Demux  Outputs=[3,3,3]
  Dot Product : DotProduct  InputSameDT=on  OutDataTypeStr=Inherit: Inherit via internal rule
  Dot Product1 : DotProduct  InputSameDT=on  OutDataTypeStr=Inherit: Inherit via internal rule
  Dot Product2 : DotProduct  InputSameDT=on  OutDataTypeStr=Inherit: Inherit via internal rule
  Gain2 : Gain  Gain=K_o  Multiplication=Matrix(K*u)  OutDataTypeStr=Inherit: Same as input  ParamDataTypeStr=Inherit: Same as input
  Mux2 : Mux  Inputs=3
  Subsystem3 : Subsystem
      mask Display: disp('2tr(E)')
  Terminator : Terminator
  Out1 : Outport
  wires:
  In1/1 -> Subsystem3/1(In1), Demux/1
  Subsystem3/1(Out1) -> Demux1/1
  Demux/2 -> Gain2/1
  Demux/1 -> Terminator/1
  Dot Product/1 -> Mux2/3
  Dot Product1/1 -> Mux2/2
  Dot Product2/1 -> Mux2/1
  Demux1/1 -> Dot Product2/1
  Demux1/2 -> Dot Product1/1
  Demux1/3 -> Dot Product/1
  Mux2/1 -> Out1/1
  Gain2/1 -> Dot Product/2, Dot Product1/2, Dot Product2/2

== system Arm_cobot/Left Arm/Impedance equation LEFT/Impedance  Equation/Subsystem1 ==
  note: angular vel.
  note: dQ_dc
  Q_dc : Inport
  w_dc : Inport  Port=2
  Mux : Mux  Inputs=[3, 4]
  S-Function : S-Function  FunctionName=Qprop_S  EnableBusSupport=off
  Out1 : Outport
  wires:
  Q_dc/1 -> Mux/2
  Mux/1 -> S-Function/1
  w_dc/1 -> Mux/1
  S-Function/1 -> Out1/1

== system Arm_cobot/Left Arm/Impedance equation LEFT/Impedance  Equation/Subsystem2 ==
  Q_2 : Inport
  Q_1 : Inport  Port=2
  Mux : Mux  Inputs=2
  S-Function : S-Function  FunctionName=Qproduct_S  EnableBusSupport=off
  Out1 : Outport
  wires:
  Q_1/1 -> Mux/1
  Q_2/1 -> Mux/2
  Mux/1 -> S-Function/1
  S-Function/1 -> Out1/1

== system Arm_cobot/Left Arm/Impedance equation LEFT/Impedance  Equation/Subsystem3 ==
  In1 : Inport
  Constant : Constant  Value=zeros(1,3)
  Switch : Switch  Threshold=.5
  Out1 : Outport
  wires:
  In1/1 -> Switch/1
  [LCpl] -> Switch/2
  Switch/1 -> Out1/1
  Constant/1 -> Switch/3

== system Arm_cobot/Left Arm/Impedance equation LEFT/Impedance  Equation/Subsystem4 ==
  In1 : Inport
  Constant : Constant  Value=zeros(1,3)
  Switch : Switch  Threshold=.5
  Out1 : Outport
  wires:
  In1/1 -> Switch/1
  [LCpl] -> Switch/2
  Switch/1 -> Out1/1
  Constant/1 -> Switch/3

== system Arm_cobot/Left Arm/Impedance equation LEFT/Impedance  Equation/Subsystem6 ==
  In1 : Inport
  Constant : Constant  Value=zeros(1,4)
  Switch : Switch  Threshold=.5
  Out1 : Outport
  wires:
  In1/1 -> Switch/1
  [LCpl] -> Switch/2
  Switch/1 -> Out1/1
  Constant/1 -> Switch/3

== system Arm_cobot/Left Arm/Impedance equation LEFT/Impedance  Equation/Subsystem7 ==
  In1 : Inport
  Constant : Constant  Value=zeros(1,3)
  Switch : Switch  Threshold=.5
  Out1 : Outport
  wires:
  In1/1 -> Switch/1
  [LCpl] -> Switch/2
  Switch/1 -> Out1/1
  Constant/1 -> Switch/3

== system Arm_cobot/Left Arm/Inverse kinematics LEFT/IK_L weighted damped least square/PID ==
  In : Inport
  D value : Gain  Gain=KdC
  Derivative : Derivative
  I value : Gain  Gain=KiC
  Integrator : Integrator
  P value : Gain  Gain=KpC
  Saturation : Saturate  UpperLimit=10  LowerLimit=-10
  Sum2 : Sum  Inputs=+++
  Out : Outport
  wires:
  Sum2/1 -> Out/1
  Derivative/1 -> D value/1
  Integrator/1 -> I value/1
  In/1 -> Derivative/1, Integrator/1, P value/1
  I value/1 -> Saturation/1
  P value/1 -> Sum2/1
  Saturation/1 -> Sum2/2
  D value/1 -> Sum2/3

== system Arm_cobot/Left Arm/Inverse kinematics LEFT/IK_L weighted damped least square/Quaternion to  angular velocity ==
  Q : Inport
  Derivative1 : Derivative
  Mux : Mux  Inputs=2
  S-Function1 : S-Function  FunctionName=Q2AngVel_S  EnableBusSupport=off
  W : Outport
  wires:
  Derivative1/1 -> Mux/2
  Mux/1 -> S-Function1/1
  Q/1 -> Derivative1/1, Mux/1
  S-Function1/1 -> W/1

== system Arm_cobot/Left Arm/Inverse kinematics LEFT/IK_L weighted damped least square/WDLS ==
  XL_dot : Inport
  qL : Inport  Port=2
  Anti Windup : MATLAB Function  TreatAsAtomicUnit=on
  Jacobian : S-Function  FunctionName=j_S  EnableBusSupport=off
  LTCP : Constant  Value=LTool_L
  Math Function : Math  Operator=transpose  SaturateOnIntegerOverflow=on
  Mux : Mux  Inputs=2
  Reshape : Reshape  OutputDimensionality=Customize  OutputDimensions=[7,7]
  WDLS left : MATLAB Function  TreatAsAtomicUnit=on
  q'2q : Integrator  InitialCondition=qIL
  q_damp : Outport
  wires:
  Mux/1 -> Jacobian/1
  LTCP/1 -> Mux/1
  qL/1 -> Mux/2, WDLS left/3(q), Anti Windup/2(q)
  Jacobian/1 -> Reshape/1
  Reshape/1 -> Math Function/1
  q'2q/1 -> q_damp/1
  Math Function/1 -> WDLS left/1(jacobian)
  XL_dot/1 -> WDLS left/2(xDot)
  WDLS left/1(qDot) -> Anti Windup/1(qDot)
  Anti Windup/1(qDot1) -> q'2q/1

== system Arm_cobot/Left Arm/Left Arm/Arms/Analog Output1 ==
  In2 : Inport
  Analog Output : sensoray/Analog Output  BoardNumber=2  Channels=[0 1 2 3]  InitialOutputs=[0 0 0 0]  FinalOutputs=[0 0 0 0]  SampleTime=-1
  Analog Output1 : sensoray/Analog Output  BoardNumber=3  Channels=[0 1 2]  InitialOutputs=[0 0 0]  FinalOutputs=[0 0 0]  SampleTime=-1
  Demux : Demux  Outputs=2
  wires:
  In2/1 -> Demux/1
  Demux/1 -> Analog Output/1
  Demux/2 -> Analog Output1/1

== system Arm_cobot/Left Arm/Left Arm/Arms/Encoder Input1 ==
  Encoder Input : sensoray/Encoder Input  BoardNumber=2  Channels=[0 2 3 5]  InitialValues=[0 0 0 0]  SampleTime=simget(bdroot,'FixedStep')  ResetEncoder=off
  Encoder Input1 : sensoray/Encoder Input  BoardNumber=3  Channels=[0 2 3]  InitialValues=[0 0 0]  SampleTime=simget(bdroot,'FixedStep')  ResetEncoder=off
  Mux : Mux  Inputs=2
  Out1 : Outport
  wires:
  Encoder Input/1 -> Mux/1
  Encoder Input1/1 -> Mux/2
  Mux/1 -> Out1/1

== system Arm_cobot/Left Arm/Left Arm/Arms/Pose A offset1 ==
  in : Inport
  Constant : Constant  Value=pi/2
  Constant1 : Constant  Value=0
  Constant2 : Constant  Value=0
  Demux : Demux  Outputs=7
  Mux : Mux  Inputs=7
  Sum : Sum  Inputs=++|  SaturateOnIntegerOverflow=on  InputSameDT=on  OutDataTypeStr=Inherit: Same as first input
  Sum1 : Sum  Inputs=++|  SaturateOnIntegerOverflow=on  InputSameDT=on  OutDataTypeStr=Inherit: Same as first input
  Sum2 : Sum  Inputs=++|  SaturateOnIntegerOverflow=on  InputSameDT=on  OutDataTypeStr=Inherit: Same as first input
  out : Outport
  wires:
  Mux/1 -> out/1
  in/1 -> Demux/1
  Demux/4 -> Mux/4
  Sum1/1 -> Mux/3
  Constant1/1 -> Sum1/1
  Demux/3 -> Sum1/2
  Sum/1 -> Mux/2
  Demux/2 -> Sum/2
  Constant/1 -> Sum/1
  Demux/1 -> Mux/1
  Demux/5 -> Mux/5
  Demux/6 -> Mux/6
  Sum2/1 -> Mux/7
  Constant2/1 -> Sum2/1
  Demux/7 -> Sum2/2

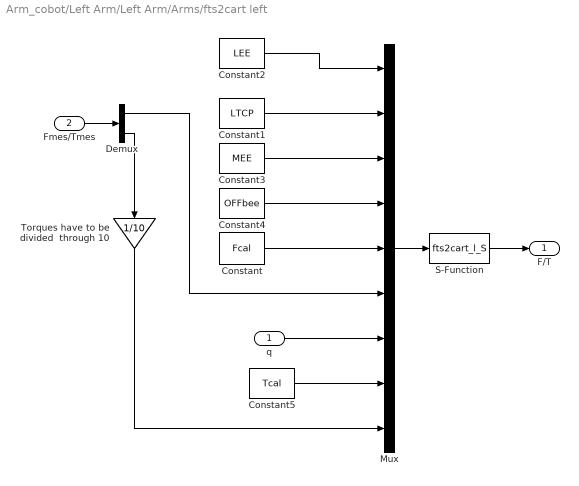
== system Arm_cobot/Left Arm/Left Arm/Arms/fts2cart left ==
  q : Inport
  Fmes/Tmes : Inport  Port=2
  Constant : Constant  Value=Fcal
  Constant1 : Constant  Value=LTCP
  Constant2 : Constant  Value=LEE
  Constant3 : Constant  Value=MEE
  Constant4 : Constant  Value=OFFbee
  Constant5 : Constant  Value=Tcal
  Demux : Demux  Outputs=2
  Mux : Mux  Inputs=9
  S-Function : S-Function  FunctionName=fts2cart_l_S  EnableBusSupport=off
  Torques have to be divided  through 10 : Gain  Gain=1/10
  F/T : Outport
  wires:
  Torques have to be divided  through 10/1 -> Mux/9
  Mux/1 -> S-Function/1
  S-Function/1 -> F/T/1
  Fmes/Tmes/1 -> Demux/1
  q/1 -> Mux/7
  Constant5/1 -> Mux/8
  Demux/2 -> Torques have to be divided  through 10/1
  Constant2/1 -> Mux/1
  Constant1/1 -> Mux/2
  Constant3/1 -> Mux/3
  Constant4/1 -> Mux/4
  Constant/1 -> Mux/5
  Demux/1 -> Mux/6

== system Arm_cobot/Left Arm/PD Joint Control  LEFT/PID Digital Derivative1/PID + digital Derivative1 ==
  In_1 : Inport
  Discrete Transfer Fcn : DiscreteTransferFcn  Numerator=[1 -1]  Denominator=TA*[1 0]  SampleTime=TA
  Integral : TransferFcn  Numerator=[I]  Denominator=[1 0]
  Proportional : Gain  Gain=P  SaturateOnIntegerOverflow=on  OutDataTypeStr=Inherit: Same as input  ParamDataTypeStr=Inherit: Same as input
  Proportional1 : Gain  Gain=D  SaturateOnIntegerOverflow=on  OutDataTypeStr=Inherit: Same as input  ParamDataTypeStr=Inherit: Same as input
  Sum : Sum  Inputs=+++  SaturateOnIntegerOverflow=on  InputSameDT=on  OutDataTypeStr=Inherit: Same as first input
  Out_1 : Outport  InitialOutput=0
  wires:
  Proportional1/1 -> Discrete Transfer Fcn/1
  Proportional/1 -> Sum/1
  Integral/1 -> Sum/2
  Discrete Transfer Fcn/1 -> Sum/3
  In_1/1 -> Proportional/1, Integral/1, Proportional1/1
  Sum/1 -> Out_1/1

== system Arm_cobot/Left Arm/PD Joint Control  LEFT/PID Digital Derivative1/PID + digital Derivative2 ==
  In_1 : Inport
  Discrete Transfer Fcn : DiscreteTransferFcn  Numerator=[1 -1]  Denominator=TA*[1 0]  SampleTime=TA
  Integral : TransferFcn  Numerator=[I]  Denominator=[1 0]
  Proportional : Gain  Gain=P  SaturateOnIntegerOverflow=on  OutDataTypeStr=Inherit: Same as input  ParamDataTypeStr=Inherit: Same as input
  Proportional1 : Gain  Gain=D  SaturateOnIntegerOverflow=on  OutDataTypeStr=Inherit: Same as input  ParamDataTypeStr=Inherit: Same as input
  Sum : Sum  Inputs=+++  SaturateOnIntegerOverflow=on  InputSameDT=on  OutDataTypeStr=Inherit: Same as first input
  Out_1 : Outport  InitialOutput=0
  wires:
  Sum/1 -> Out_1/1
  In_1/1 -> Proportional1/1, Integral/1, Proportional/1
  Discrete Transfer Fcn/1 -> Sum/3
  Integral/1 -> Sum/2
  Proportional/1 -> Sum/1
  Proportional1/1 -> Discrete Transfer Fcn/1

== system Arm_cobot/Left Arm/PD Joint Control  LEFT/PID Digital Derivative1/PID + digital Derivative3 ==
  In_1 : Inport
  Discrete Transfer Fcn : DiscreteTransferFcn  Numerator=[1 -1]  Denominator=TA*[1 0]  SampleTime=TA
  Integral : TransferFcn  Numerator=[I]  Denominator=[1 0]
  Proportional : Gain  Gain=P  SaturateOnIntegerOverflow=on  OutDataTypeStr=Inherit: Same as input  ParamDataTypeStr=Inherit: Same as input
  Proportional1 : Gain  Gain=D  SaturateOnIntegerOverflow=on  OutDataTypeStr=Inherit: Same as input  ParamDataTypeStr=Inherit: Same as input
  Sum : Sum  Inputs=+++  SaturateOnIntegerOverflow=on  InputSameDT=on  OutDataTypeStr=Inherit: Same as first input
  Out_1 : Outport  InitialOutput=0
  wires:
  Sum/1 -> Out_1/1
  In_1/1 -> Proportional1/1, Integral/1, Proportional/1
  Discrete Transfer Fcn/1 -> Sum/3
  Integral/1 -> Sum/2
  Proportional/1 -> Sum/1
  Proportional1/1 -> Discrete Transfer Fcn/1

== system Arm_cobot/Left Arm/PD Joint Control  LEFT/PID Digital Derivative1/PID + digital Derivative4 ==
  In_1 : Inport
  Discrete Transfer Fcn : DiscreteTransferFcn  Numerator=[1 -1]  Denominator=TA*[1 0]  SampleTime=TA
  Integral : TransferFcn  Numerator=[I]  Denominator=[1 0]
  Proportional : Gain  Gain=P  SaturateOnIntegerOverflow=on  OutDataTypeStr=Inherit: Same as input  ParamDataTypeStr=Inherit: Same as input
  Proportional1 : Gain  Gain=D  SaturateOnIntegerOverflow=on  OutDataTypeStr=Inherit: Same as input  ParamDataTypeStr=Inherit: Same as input
  Sum : Sum  Inputs=+++  SaturateOnIntegerOverflow=on  InputSameDT=on  OutDataTypeStr=Inherit: Same as first input
  Out_1 : Outport  InitialOutput=0
  wires:
  Proportional1/1 -> Discrete Transfer Fcn/1
  Proportional/1 -> Sum/1
  Integral/1 -> Sum/2
  Discrete Transfer Fcn/1 -> Sum/3
  In_1/1 -> Proportional/1, Integral/1, Proportional1/1
  Sum/1 -> Out_1/1

== system Arm_cobot/Left Arm/PD Joint Control  LEFT/PID Digital Derivative1/PID + digital Derivative5 ==
  In_1 : Inport
  Discrete Transfer Fcn : DiscreteTransferFcn  Numerator=[1 -1]  Denominator=TA*[1 0]  SampleTime=TA
  Integral : TransferFcn  Numerator=[I]  Denominator=[1 0]
  Proportional : Gain  Gain=P  SaturateOnIntegerOverflow=on  OutDataTypeStr=Inherit: Same as input  ParamDataTypeStr=Inherit: Same as input
  Proportional1 : Gain  Gain=D  SaturateOnIntegerOverflow=on  OutDataTypeStr=Inherit: Same as input  ParamDataTypeStr=Inherit: Same as input
  Sum : Sum  Inputs=+++  SaturateOnIntegerOverflow=on  InputSameDT=on  OutDataTypeStr=Inherit: Same as first input
  Out_1 : Outport  InitialOutput=0
  wires:
  Sum/1 -> Out_1/1
  In_1/1 -> Proportional1/1, Integral/1, Proportional/1
  Discrete Transfer Fcn/1 -> Sum/3
  Integral/1 -> Sum/2
  Proportional/1 -> Sum/1
  Proportional1/1 -> Discrete Transfer Fcn/1

== system Arm_cobot/Left Arm/PD Joint Control  LEFT/PID Digital Derivative1/PID + digital Derivative6 ==
  In_1 : Inport
  Discrete Transfer Fcn : DiscreteTransferFcn  Numerator=[1 -1]  Denominator=TA*[1 0]  SampleTime=TA
  Integral : TransferFcn  Numerator=[I]  Denominator=[1 0]
  Proportional : Gain  Gain=P  SaturateOnIntegerOverflow=on  OutDataTypeStr=Inherit: Same as input  ParamDataTypeStr=Inherit: Same as input
  Proportional1 : Gain  Gain=D  SaturateOnIntegerOverflow=on  OutDataTypeStr=Inherit: Same as input  ParamDataTypeStr=Inherit: Same as input
  Sum : Sum  Inputs=+++  SaturateOnIntegerOverflow=on  InputSameDT=on  OutDataTypeStr=Inherit: Same as first input
  Out_1 : Outport  InitialOutput=0
  wires:
  Proportional1/1 -> Discrete Transfer Fcn/1
  Proportional/1 -> Sum/1
  Integral/1 -> Sum/2
  Discrete Transfer Fcn/1 -> Sum/3
  In_1/1 -> Proportional/1, Integral/1, Proportional1/1
  Sum/1 -> Out_1/1

== system Arm_cobot/Left Arm/PD Joint Control  LEFT/PID Digital Derivative1/PID + digital Derivative7 ==
  In_1 : Inport
  Discrete Transfer Fcn : DiscreteTransferFcn  Numerator=[1 -1]  Denominator=TA*[1 0]  SampleTime=TA
  Integral : TransferFcn  Numerator=[I]  Denominator=[1 0]
  Proportional : Gain  Gain=P  SaturateOnIntegerOverflow=on  OutDataTypeStr=Inherit: Same as input  ParamDataTypeStr=Inherit: Same as input
  Proportional1 : Gain  Gain=D  SaturateOnIntegerOverflow=on  OutDataTypeStr=Inherit: Same as input  ParamDataTypeStr=Inherit: Same as input
  Sum : Sum  Inputs=+++  SaturateOnIntegerOverflow=on  InputSameDT=on  OutDataTypeStr=Inherit: Same as first input
  Out_1 : Outport  InitialOutput=0
  wires:
  Sum/1 -> Out_1/1
  In_1/1 -> Proportional1/1, Integral/1, Proportional/1
  Discrete Transfer Fcn/1 -> Sum/3
  Integral/1 -> Sum/2
  Proportional/1 -> Sum/1
  Proportional1/1 -> Discrete Transfer Fcn/1

== system Arm_cobot/Right Arm/ForceControl/Subsystem/PII ==
  In_1 : Inport
  reset : Inport  Port=2
  Integrator : Integrator  ExternalReset=falling  UpperSaturationLimit=S  LowerSaturationLimit=-S
  Proportional : Gain  Gain=P  SaturateOnIntegerOverflow=on  OutDataTypeStr=Inherit: Same as input  ParamDataTypeStr=Inherit: Same as input
  Saturation : Saturate  UpperLimit=S  LowerLimit=-S
  Sum : Sum  SaturateOnIntegerOverflow=on  InputSameDT=on  OutDataTypeStr=Inherit: Same as first input
  Sum1 : Sum  Inputs=-+|
  Sum2 : Sum  Inputs=|++
  Out_1 : Outport  InitialOutput=0
  wires:
  Proportional/1 -> Sum/1
  Integrator/1 -> Sum/2
  Sum/1 -> Sum1/1, Saturation/1
  Sum2/1 -> Integrator/1
  In_1/1 -> Sum2/1, Proportional/1
  Saturation/1 -> Sum1/2, Out_1/1
  Sum1/1 -> Sum2/2
  reset/1 -> Integrator/2

== system Arm_cobot/Right Arm/ForceControl/Subsystem/PII1 ==
  In_1 : Inport
  reset : Inport  Port=2
  Integrator : Integrator  ExternalReset=falling  UpperSaturationLimit=S  LowerSaturationLimit=-S
  Proportional : Gain  Gain=P  SaturateOnIntegerOverflow=on  OutDataTypeStr=Inherit: Same as input  ParamDataTypeStr=Inherit: Same as input
  Saturation : Saturate  UpperLimit=S  LowerLimit=-S
  Sum : Sum  SaturateOnIntegerOverflow=on  InputSameDT=on  OutDataTypeStr=Inherit: Same as first input
  Sum1 : Sum  Inputs=-+|
  Sum2 : Sum  Inputs=|++
  Out_1 : Outport  InitialOutput=0
  wires:
  Proportional/1 -> Sum/1
  Integrator/1 -> Sum/2
  Sum/1 -> Sum1/1, Saturation/1
  Sum2/1 -> Integrator/1
  In_1/1 -> Sum2/1, Proportional/1
  Saturation/1 -> Sum1/2, Out_1/1
  Sum1/1 -> Sum2/2
  reset/1 -> Integrator/2
